simulink model "LaneTracking"  (R2023b)
settings: Solver=VariableStepAuto  StartTime=0.0  StopTime=Te  RelTol=1e-3
values from neighbouring files (symbols this model uses):
  Ts = 0.1    [ScriptBoot.m]    (also in ScriptBoot_TEST.m)
undefined symbols (not defined in the file or in its folder): driving, egoCarID, targetSpeed
libraries: drivingscenarioandsensors x7, robotcorelib x2, sensorinslib x1
(part 1 of 3)
settings Model: NumberOfSteps=10  SnapshotBufferSize=1000  SnapshotInterval=100  Creator=Victor  LastModifiedBy=Victor
settings RTWCC: Toolchain=MinGW64 | CMake/gmake (64-bit Windows)  BuildConfiguration=Release

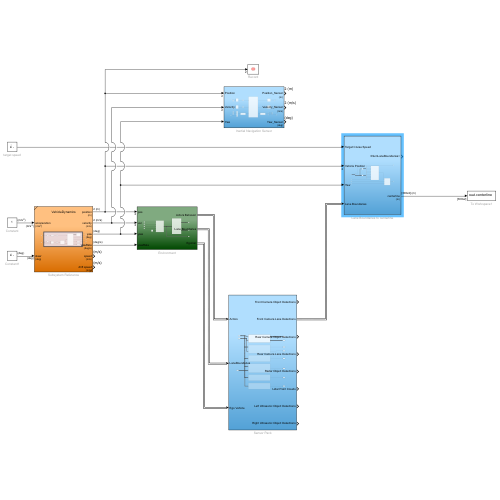
[thumbnail: Simulink's stored preview of the top-level diagram]
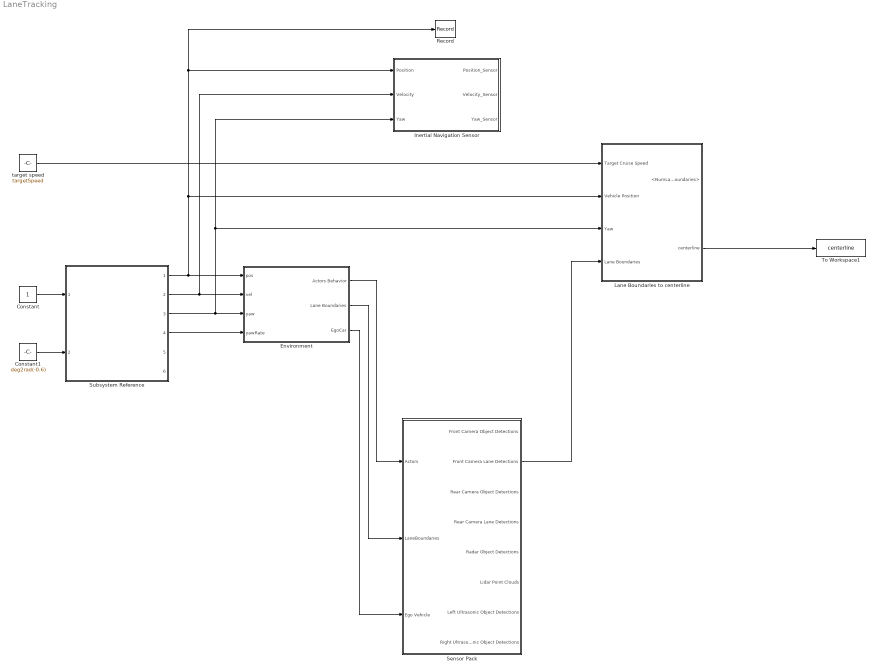
== system LaneTracking ==
  Constant : Constant
  Constant1 : Constant  Value=deg2rad(-0.6)
  Environment : Subsystem
  Inertial Navigation Sensor : Subsystem
  Lane Boundaries to centerline : Subsystem
  Record : Record  FileSettingsInternal="{\"entries\":[{\"content\":{\"excelSettings\":{\"content\":{},\"type\":\"Streamout.ExcelSettings\"}},\"type\":\"Streamout.FileSettingStorage\",\"uuid\":\"\"}],\"packageUris\":[\"http:\\/\\/schema.mathworks.com\\/mf0\\/streamout_blocks\\/R2020a\"],\"version\":\"1.0\"}"  Layout=[1 1]  SignalsInternal="{\"entries\":[{\"content\":{\"signals\":[{\"content\":{\"blockPath\":[],\"dimensions\":[2],\"domain\":\"\",\"hasChildren\":true,\"lineColor\":\"#edb120\",\"port\":1,\"sid\":[\"\"],\"signalID\":24074,\"signalName\":\"Subsystem Reference:1\"},\"type\":\"RecordBlkView.Signal\",\"uuid\":\"\"},{\"content\":{\"blockPath\":[],\"channel\":[1],\"dimensions\":[2],\"domain\":\"\",\"lineColor\":\"#7e2f8e\",\"parentID\":24074,\"plots\":[1],\"port\":1,\"sid\":[\"\"],\"signalID\":24075,\"signalName\":\"Subsystem Reference:1\"},\"type\":\"RecordBlkView.Signal\",\"uuid\":\"\"},{\"content\":{\"blockPath\":[],\"channel\":[2],\"dimensions\":[2],\"domain\":\"\",\"lineColor\":\"#b746ff\",\"parentID\":24074,\"plots\":[1],\"port\":1,\"sid\":[\"\"],\"signalID\":26031,\"signalName\":\"Subsystem Reference:1\"},\"type\":\"RecordBlkView.Signal\",\"uuid\":\"\"}]},\"type\":\"RecordBlkView.InputSignals\",\"uuid\":\"\"}],\"packageUris\":[\"http:\\/\\/schema.mathworks.com\\/mf0\\/streamout_blocks\\/R2020a\"],\"version\":\"1.0\"}"  VisualizationBindings="{\"xyplotplugin\":{\"info\":[{\"series\":[{\"bindingParametersList\":[{\"parameter\":\"X-Axis\",\"signalID\":24075,\"signalName\":\"Subsystem Reference:1(1)\"},{\"parameter\":\"Y-Axis\",\"signalID\":26031,\"signalName\":\"Subsystem Reference:1(2)\"}],\"seriesID\":29061}],\"subplotID\":1}]}}"
  Sensor Pack : Subsystem
  Subsystem Reference : Subsystem  ReferencedSubsystem=VehicleDynamics
  To Workspace1 : ToWorkspace  VariableName=centerline  SaveFormat=Timeseries  SampleTime=Ts
  target speed : Constant  Value=targetSpeed
  wires:
  Constant/1 -> Subsystem Reference/1
  Constant1/1 -> Subsystem Reference/2
  Subsystem Reference/1 -> Environment/1(pos), Record/1, Inertial Navigation Sensor/1(Position), Lane Boundaries to centerline/2(Vehicle Position)
  Subsystem Reference/2 -> Inertial Navigation Sensor/2(Velocity), Environment/2(vel)
  Subsystem Reference/3 -> Inertial Navigation Sensor/3(Yaw), Lane Boundaries to centerline/3(Yaw), Environment/3(yaw)
  Subsystem Reference/4 -> Environment/4(yawRate)
  Environment/1(Actors Behavior) -> Sensor Pack/1(Actors)
  Environment/2(Lane Boundaries) -> Sensor Pack/2(LaneBoundaries)
  Environment/3(EgoCar) -> Sensor Pack/3(Ego Vehicle)
  Sensor Pack/2(Front Camera Lane Detections) -> Lane Boundaries to centerline/4(Lane Boundaries)
  target speed/1 -> Lane Boundaries to centerline/1(Target Cruise Speed)
  Lane Boundaries to centerline/2(centerline) -> To Workspace1/1

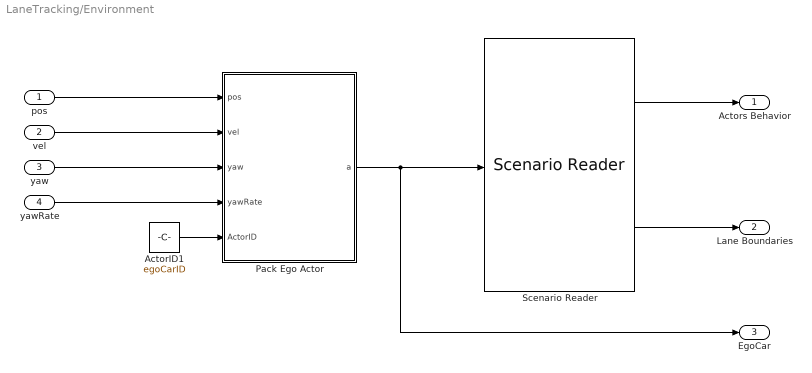
== system LaneTracking/Environment ==
  pos : Inport
  vel : Inport  Port=2
  yaw : Inport  Port=3
  yawRate : Inport  Port=4
  ActorID1 : Constant  Value=egoCarID
  Pack Ego Actor : MATLAB Function  TreatAsAtomicUnit=on
  Scenario Reader : drivingscenarioandsensors/Scenario Reader  ScenarioSource=From file  ScenarioFileName=Scenario_OneEgoCar.mat  ScenarioVariableName=scenario  OutputCoordinateSystem=Vehicle coordinates  EgoVehicleSource=Input port  EgoVehicleActorID=egoCarID  OrientVehiclesOnRoad=on  OutputEgoVehiclePose=off  OutputEgoVehicleState=off  SampleTime=Ts  LaneBoundaryOutput=Ego vehicle lane boundaries  LaneBoundaryDistance=0:0.5:60  LaneBoundaryLocation=Inner edge of lane markings  BusNameSource=Auto  BusName=BusActorsActors  BusNumActorsSource=Scenario  BusNumActors=100  BusName2Source=Auto  BusName2=BusLaneBoundaries  BusNumLaneBoundariesSource=Scenario  BusNumLaneBoundaries=10  BusName3Source=Auto  BusName3=BusEgoActor  BusName4Source=Auto  BusName4=BusEgoState  ShowCoordinateLabels=on  SimulateUsing=Code generation
  Actors Behavior : Outport
  Lane Boundaries : Outport  Port=2
  EgoCar : Outport  Port=3
  wires:
  pos/1 -> Pack Ego Actor/1(pos)
  Pack Ego Actor/1(a) -> Scenario Reader/1, EgoCar/1
  ActorID1/1 -> Pack Ego Actor/5(ActorID)
  Scenario Reader/1 -> Actors Behavior/1
  vel/1 -> Pack Ego Actor/2(vel)
  yaw/1 -> Pack Ego Actor/3(yaw)
  yawRate/1 -> Pack Ego Actor/4(yawRate)
  Scenario Reader/2 -> Lane Boundaries/1

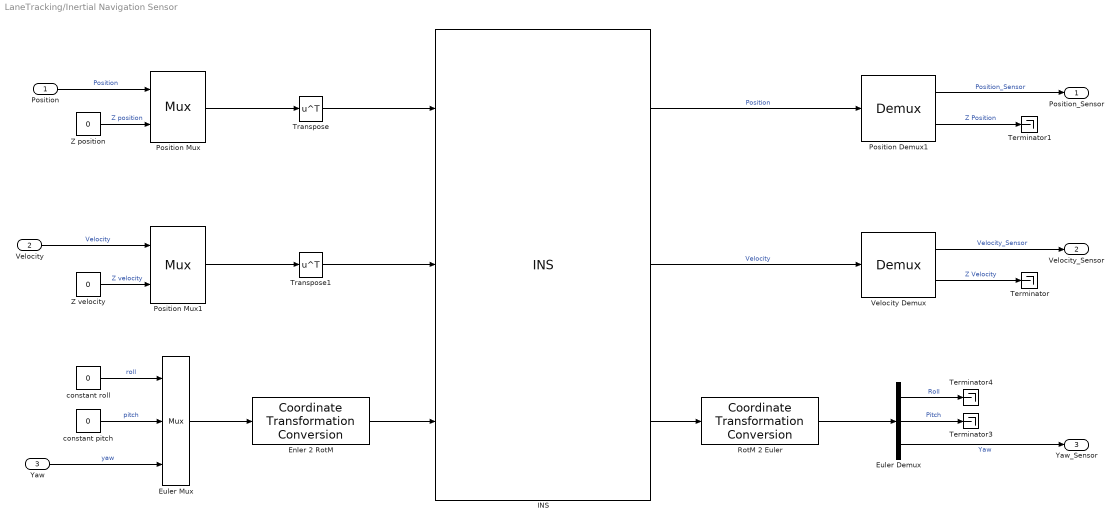
== system LaneTracking/Inertial Navigation Sensor ==
  Position : Inport
  Velocity : Inport  Port=2
  Yaw : Inport  Port=3
  Enler 2 RotM : robotcorelib/Coordinate Transformation Conversion  InputRepresentation=Euler Angles  InputEulerSequence=XYZ  ShowTrVecInputPort=on  OutputRepresentation=Rotation Matrix  OutputEulerSequence=XYZ  ShowTrVecOutputPort=on  SimulateUsing=Code generation
      settings: LibrarySourceBlock=uavutilslib/Coordinate Transformation Conversion
  Euler Demux : Demux  Outputs=3
      settings: DisplayOption=none
  Euler Mux : Mux  Inputs=3
      settings: DisplayOption=signals
  INS : sensorinslib/INS  MountingLocation=[0 0 0]  RollAccuracy=angleAccuraccy  PitchAccuracy=angleAccuraccy  YawAccuracy=angleAccuraccy  PositionAccuracy=positionAccuracy  VelocityAccuracy=velocityAccuracy  UseAccelAndAngVel=off  AccelerationAccuracy=0  AngularVelocityAccuracy=0  TimeInput=off  PositionErrorFactor=[0 0 0]  SeedDouble=32  SimulateUsing=Code generation
      settings: LibrarySourceBlock=drivingscenarioandsensors/INS
  Position Demux1 : Demux  Outputs=2
      settings: DisplayOption=none
  Position Mux : Mux  Inputs=2
      settings: DisplayOption=signals
  Position Mux1 : Mux  Inputs=2
      settings: DisplayOption=signals
  RotM 2 Euler : robotcorelib/Coordinate Transformation Conversion  InputRepresentation=Rotation Matrix  InputEulerSequence=XYZ  ShowTrVecInputPort=on  OutputRepresentation=Euler Angles  OutputEulerSequence=XYZ  ShowTrVecOutputPort=on  SimulateUsing=Code generation
      settings: LibrarySourceBlock=uavutilslib/Coordinate Transformation Conversion
  Terminator{,1,3..4} (4 alike) : Terminator
  Transpose : Math  Operator=transpose
  Transpose1 : Math  Operator=transpose
  Velocity Demux : Demux  Outputs=2
      settings: DisplayOption=none
  Z position : Constant  Value=0
  Z velocity : Constant  Value=0
  constant pitch : Constant  Value=0
  constant roll : Constant  Value=0
  Position_Sensor : Outport  Unit=m  PortDimensions=2
  Velocity_Sensor : Outport  Port=2  Unit=m/s  PortDimensions=2
  Yaw_Sensor : Outport  Port=3  Unit=deg
  wires:
  Enler 2 RotM/1 -> INS/3
  Euler Demux/1 -> Terminator4/1  "Roll"
  Euler Mux/1 -> Enler 2 RotM/1
  RotM 2 Euler/1 -> Euler Demux/1
  Euler Demux/3 -> Yaw_Sensor/1  "Yaw"
  INS/3 -> RotM 2 Euler/1
  Euler Demux/2 -> Terminator3/1  "Pitch"
  constant roll/1 -> Euler Mux/1  "roll"
  constant pitch/1 -> Euler Mux/2  "pitch"
  Yaw/1 -> Euler Mux/3  "yaw"
  Position/1 -> Position Mux/1  "Position"
  Z position/1 -> Position Mux/2  "Z position"
  Z velocity/1 -> Position Mux1/2  "Z velocity"
  Velocity/1 -> Position Mux1/1  "Velocity"
  Position Mux/1 -> Transpose/1
  Transpose/1 -> INS/1
  Position Mux1/1 -> Transpose1/1
  Transpose1/1 -> INS/2
  INS/2 -> Velocity Demux/1  "Velocity"
  Velocity Demux/1 -> Velocity_Sensor/1  "Velocity_Sensor"
  Velocity Demux/2 -> Terminator/1  "Z Velocity"
  Position Demux1/1 -> Position_Sensor/1  "Position_Sensor"
  Position Demux1/2 -> Terminator1/1  "Z Position"
  INS/1 -> Position Demux1/1  "Position"

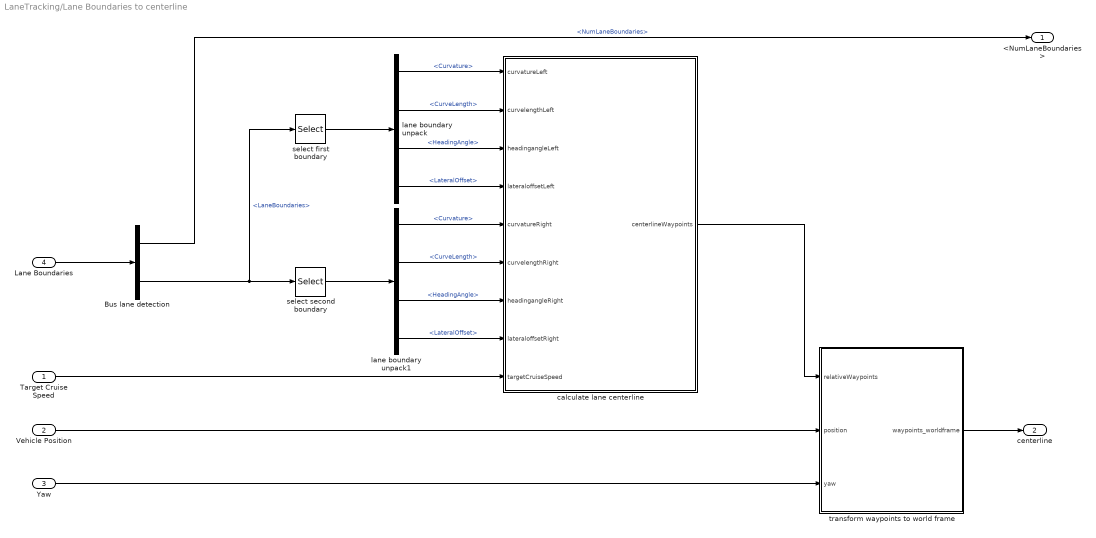
== system LaneTracking/Lane Boundaries to centerline ==
  Target Cruise Speed : Inport
  Vehicle Position : Inport  Port=2
  Yaw : Inport  Port=3
  Lane Boundaries : Inport  Port=4
  Bus lane detection : BusSelector  OutputSignals=NumLaneBoundaries,LaneBoundaries
  "calculate lane centerline " : MATLAB Function  TreatAsAtomicUnit=on
  lane boundary unpack : BusSelector  OutputSignals=Curvature,CurveLength,HeadingAngle,LateralOffset
  lane boundary unpack1 : BusSelector  OutputSignals=Curvature,CurveLength,HeadingAngle,LateralOffset
  select first boundary : Selector  InputPortWidth=4  IndexOptions=Index vector (dialog)  Indices=[1]  OutputSizes=1
  select second boundary : Selector  InputPortWidth=4  IndexOptions=Index vector (dialog)  Indices=[2]  OutputSizes=1
  transform waypoints to world frame : MATLAB Function  TreatAsAtomicUnit=on
  <NumLaneBoundaries> : Outport
  centerline : Outport  Port=2  Unit=m
  wires:
  lane boundary unpack1/3 -> "calculate lane centerline "/7(headingangleRight)  "<HeadingAngle>"
  select first boundary/1 -> lane boundary unpack/1
  lane boundary unpack/4 -> "calculate lane centerline "/4(lateraloffsetLeft)  "<LateralOffset>"
  lane boundary unpack/2 -> "calculate lane centerline "/2(curvelengthLeft)  "<CurveLength>"
  Bus lane detection/2 -> select second boundary/1, select first boundary/1  "<LaneBoundaries>"
  lane boundary unpack1/1 -> "calculate lane centerline "/5(curvatureRight)  "<Curvature>"
  lane boundary unpack1/4 -> "calculate lane centerline "/8(lateraloffsetRight)  "<LateralOffset>"
  select second boundary/1 -> lane boundary unpack1/1
  lane boundary unpack1/2 -> "calculate lane centerline "/6(curvelengthRight)  "<CurveLength>"
  lane boundary unpack/3 -> "calculate lane centerline "/3(headingangleLeft)  "<HeadingAngle>"
  lane boundary unpack/1 -> "calculate lane centerline "/1(curvatureLeft)  "<Curvature>"
  Target Cruise Speed/1 -> "calculate lane centerline "/9(targetCruiseSpeed)
  Bus lane detection/1 -> <NumLaneBoundaries>/1  "<NumLaneBoundaries>"
  Lane Boundaries/1 -> Bus lane detection/1
  Vehicle Position/1 -> transform waypoints to world frame/2(position)
  Yaw/1 -> transform waypoints to world frame/3(yaw)
  transform waypoints to world frame/1(waypoints_worldframe) -> centerline/1
  "calculate lane centerline "/1(centerlineWaypoints) -> transform waypoints to world frame/1(relativeWaypoints)
